simulink model "testingRocketPositionControl"  (R2020a)
settings: Solver=ode4  StartTime=0.0  StopTime=50  FixedStep=0.001  RelTol=1e-3
undefined symbols (not defined in the file): g, I, K_aug, L, m
settings Model: Creator=Amir  LastModifiedBy=Flaz
settings DataIOCC: ReturnWorkspaceOutputs=off
settings DebuggingCC: ArithmeticOperatorsInVariantConditions=warning
settings SFSimCC: CustomCodeUndefinedFunction=UseInterfaceOnly

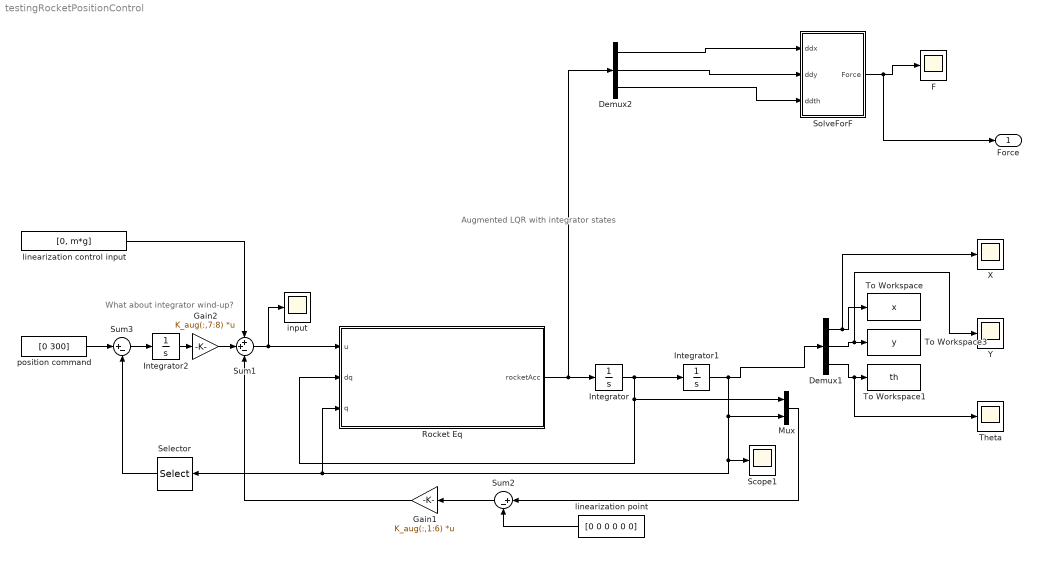
== system testingRocketPositionControl ==
  note: Augmented LQR with integrator states
  note: What about integrator wind-up?
  Demux1 : Demux  Outputs=3
  Demux2 : Demux  Outputs=3
  F : Scope
  Gain1 : Gain  Gain=K_aug(:,1:6)  Multiplication=Matrix(K*u)
  Gain2 : Gain  Gain=K_aug(:,7:8)  Multiplication=Matrix(K*u)
  Integrator : Integrator  InitialCondition=[0 0 0]
  Integrator1 : Integrator  InitialCondition=[0, 0, 0]
  Integrator2 : Integrator
  Mux : Mux  Inputs=2
  Rocket Eq : MATLAB Function  TreatAsAtomicUnit=on
  Scope1 : Scope
  Selector : Selector  InputPortWidth=3  IndexOptions=Index vector (dialog)  Indices=[1 2]  OutputSizes=1
  SolveForF : MATLAB Function  TreatAsAtomicUnit=on
  Sum1 : Sum  Inputs=++-
  Sum2 : Sum  Inputs=|+-
  Sum3 : Sum  Inputs=|+-
  Theta : Scope
  To Workspace : ToWorkspace  VariableName=x  SampleTime=0.01
  To Workspace1 : ToWorkspace  VariableName=th  SampleTime=0.01
  To Workspace3 : ToWorkspace  VariableName=y  SampleTime=0.01
  X : Scope
  Y : Scope
  input : Scope
  linearization control input : Constant  Value=[0, m*g]
  linearization point : Constant  Value=[0 0 0 0 0 0]
  position command : Constant  Value=[0 300]
  Force : Outport
  wires:
  Rocket Eq/1(rocketAcc) -> Demux2/1, Integrator/1
  Integrator/1 -> Integrator1/1, Mux/1, Rocket Eq/2(dq)
  Integrator1/1 -> Demux1/1, Mux/2, Scope1/1, Rocket Eq/3(q), Selector/1
  Sum1/1 -> input/1, Rocket Eq/1(u)
  Sum2/1 -> Gain1/1
  linearization point/1 -> Sum2/2
  Mux/1 -> Sum2/1
  linearization control input/1 -> Sum1/1
  Gain1/1 -> Sum1/3
  Integrator2/1 -> Gain2/1
  Gain2/1 -> Sum1/2
  Sum3/1 -> Integrator2/1
  position command/1 -> Sum3/1
  Selector/1 -> Sum3/2
  Demux1/1 -> X/1, To Workspace/1
  Demux1/2 -> Y/1, To Workspace3/1
  Demux1/3 -> Theta/1, To Workspace1/1
  Demux2/1 -> SolveForF/1(ddx)
  Demux2/2 -> SolveForF/2(ddy)
  Demux2/3 -> SolveForF/3(ddth)
  SolveForF/1(Force) -> Force/1, F/1

== matlab function testingRocketPositionControl/SolveForF ==
  data: ddx input; Force output; ddy input; ddth input
function Force = fcn(ddx, ddy, ddth)
%ddx = -(Fx*cos(th) + Fy*sin(th))/mass
%ddy = -(g*mass - Fy*cos(th) + Fx*sin(th))/mass
%ddth = -(7*Fx)/(2*inertia)
%Fx = -F*sin(alpha+th)
%Fy = F*cos(alpha+th)
g = 9.81;
inertia = 36833.3333333333;
mass = 1000;
F = mass*sqrt(ddx^2+ddy^2+2*ddy*g+g^2);
alpha = asin((ddx*mass)/F)

Force = F;

== matlab function testingRocketPositionControl/Rocket Eq ==
  data: u input; rocketAcc output; dq input; q input; m parameter; I parameter; L parameter; g parameter
function rocketAcc = fullDyn(u,dq,q, m, I, L, g)


Fx = u(1);
Fy = u(2);
mass = m
inertia = I;
x = q(1);
y = q(2);
th = q(3);

dx = dq(1);
dy = dq(2);
dth = dq(3);


rocketAcc = [-(Fx*cos(th) + Fy*sin(th))/mass;-(g*mass - Fy*cos(th) + Fx*sin(th))/mass;-(7*Fx)/(2*inertia)];
